simulink model "simulation"  (R2018a)
settings: Solver=VariableStepAuto  StartTime=0.0  StopTime=5  RelTol=1e-3
undefined symbols (not defined in the file): A, B, C
settings Model: Creator=Migue  LastModifiedBy=Miguel Faggioni

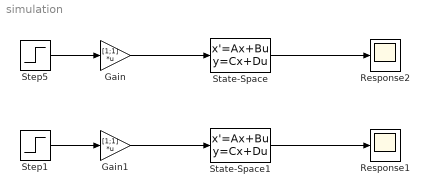
== system simulation ==
  Gain : Gain  Gain=[1;1]  Multiplication=Matrix(K*u)
  Gain1 : Gain  Gain=[1;1]  Multiplication=Matrix(K*u)
  Response1 : Scope
  Response2 : Scope
  State-Space : StateSpace  A=A  B=B  C=C  D=[0 0;0 0]  InitialCondition=0
  State-Space1 : StateSpace  A=A  B=B  C=C  D=[0 0;0 0]  InitialCondition=0
  Step1 : Step  SampleTime=0
  Step5 : Step  SampleTime=0
  wires:
  State-Space/1 -> Response2/1
  Step5/1 -> Gain/1
  Gain/1 -> State-Space/1
  Step1/1 -> Gain1/1
  Gain1/1 -> State-Space1/1
  State-Space1/1 -> Response1/1
